simulink model "chapter1_jd"  (R2016b)
settings: Solver=VariableStepAuto  StartTime=0.0  StopTime=10  RelTol=1e-3
PreLoadFcn:
  | t = linspace(0,10,101)';
  | u = linspace(0,pi/2,101)';
  | degConv = 180/pi;
settings Model: Creator=training-ah  LastModifiedBy=training-ah
settings DataIOCC: LoadExternalInput=on  SaveFormat=Array

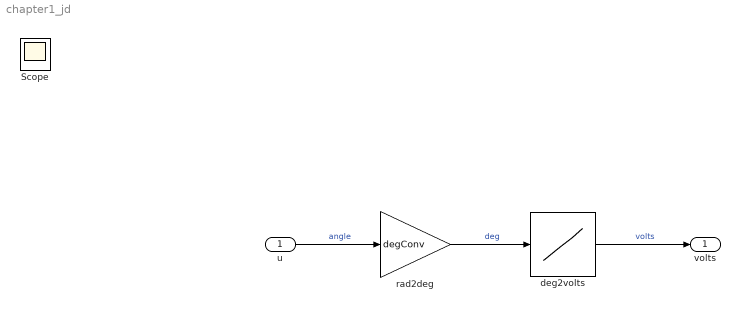
== system chapter1_jd ==
  u : Inport
  deg2volts : Lookup_n-D  NumberOfTableDimensions=1  BreakpointsForDimension1=[0 90]  Table=[0.5 4.5]  ExtrapMethod=Clip  UseLastTableValue=on  InternalRulePriority=Speed  RndMeth=Simplest  InputSameDT=on
  rad2deg : Gain  Gain=degConv
  volts : Outport
  Scope : Scope
  wires:
  u/1 -> rad2deg/1  "angle"
  rad2deg/1 -> deg2volts/1  "deg"
  deg2volts/1 -> volts/1  "volts"
